simulink model "GRM_HIL"  (R2019b)
settings: Solver=FixedStepAuto  StartTime=0.0  StopTime=60  FixedStep=0.001  RelTol=1e-3
libraries: lib_GRM_HIL x7, simulink x1
settings Model: SimulationMode=external  Creator=m.hiepp  LastModifiedBy=guy-m
settings DataIOCC: SignalLogging=off  ReturnWorkspaceOutputs=off
settings DebuggingCC: ArithmeticOperatorsInVariantConditions=warning
settings SFSimCC: CustomCodeUndefinedFunction=UseInterfaceOnly
settings RTWCC: Description=Simulink Desktop Real-Time  SystemTargetFile=sldrt.tlc  TemplateMakefile=sldrt.tmf  RTWCompilerOptimization=on
settings CodeAppCC: MaxIdLength=95
settings SimulinkDesktopRealTimeCC: TargetPreCompLibLocation=C:\Program Files\MATLAB\R2019b\toolbox\sldrt\lib\win64  PreserveStateflowLocalDataDimensions=off

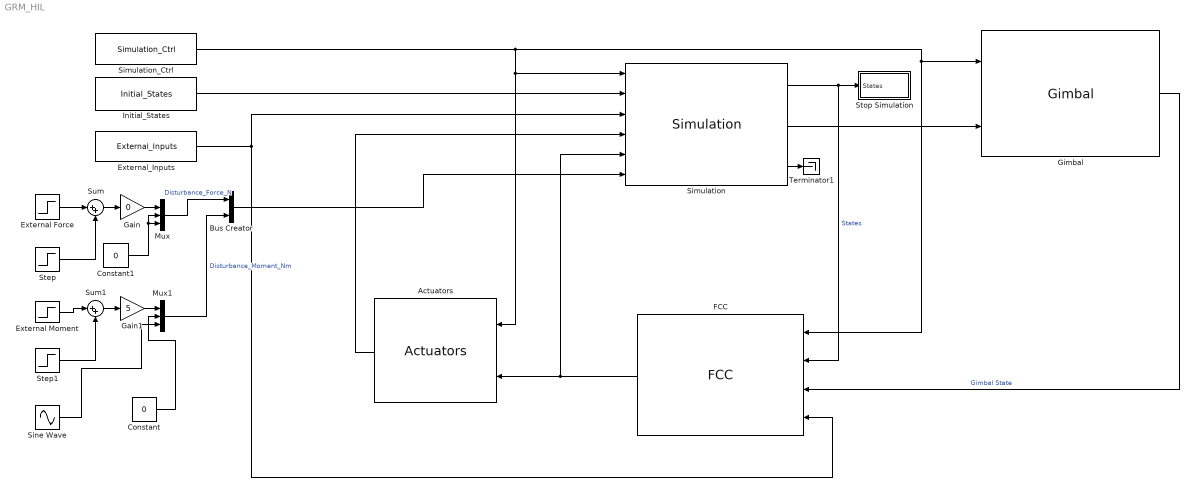
== system GRM_HIL ==
  Actuators : lib_GRM_HIL/Actuators  SystemSampleTime=-1  Latency=0  AutoFrameSizeCalculation=off
  Bus Creator : BusCreator  Inputs=2  OutDataTypeStr=Bus: Disturbances_Bus
  Constant : Constant  Value=0
  Constant1 : Constant  Value=0
  External Force : Step  Time=0  SampleTime=0
  External Moment : Step  Time=5  SampleTime=0
  External_Inputs : lib_GRM_HIL/External_Inputs  External_Inputs=HIL_Data.External_Inputs
  FCC : lib_GRM_HIL/FCC  SystemSampleTime=-1  Latency=0  AutoFrameSizeCalculation=off
      link override Use_FCC/Serial_Config_Pixhawk/enable_serial_config/Serial Configuration: ComPortMenu=COM4  BaudRate=115200  StopBits=1  ComPort=COM4  ObjConstructor=serial('COM4');
      link override Use_FCC/Serial_Recieve_from_Pixhawk/Receive_ExternalMode/Packet Input: SampleTime=HIL_Sample_Time  MaxMissedTicks=Serial.Receive.MaxMissedTicks  ShowMissedTicks=off  YieldWhenWaiting=on  DrvName=Standard_Devices/Serial_Port  DrvAddress=4  DrvOptions=[115200 8 0 0 0 0 0 0]  PacketSize=62  DataTypes='62*uint8'  ShowReady=on  ShowError=on  PacketID=1  ByteOrder=1  ShowTimestamp=off
      link override Use_FCC/Serial_Recieve_from_Pixhawk/Receive_NormalMode/Serial Configuration: ComPortMenu=COM4  BaudRate=115200  StopBits=1  ComPort=COM4  ObjConstructor=serial('COM4');
      link override Use_FCC/Serial_Recieve_from_Pixhawk/Receive_NormalMode/Serial Receive1: ComPortMenu=COM4  ComPort=COM4  ObjConstructor=serial('COM4');
      link override Use_FCC/Serial_Send_to_Pixhawk/send_to_pix/Send_ExternalMode/Packet Output: SampleTime=1/HIL_Data.Simulation_Ctrl.Com_Ctrl.Pix.Com_freq_Hz  MaxMissedTicks=Serial.Send.MaxMissedTicks  ShowMissedTicks=off  YieldWhenWaiting=on  DrvName=Standard_Devices/Serial_Port  DrvAddress=4  DrvOptions=[115200 8 0 0 0 0 0 0]  PacketSize=128  DataTypes='128*uint8'  ShowReady=off  ShowError=on  PacketID=1  ByteOrder=1  InitialValue=[]  FinalValue=[]
      link override Use_FCC/Serial_Send_to_Pixhawk/send_to_pix/Send_NormalMode/Packet Output: SampleTime=1/HIL_Data.Simulation_Ctrl.Com_Ctrl.Pix.Com_freq_Hz  MaxMissedTicks=Serial.Send.MaxMissedTicks  ShowMissedTicks=off  YieldWhenWaiting=on  DrvName=Standard_Devices/Serial_Port  DrvAddress=1  DrvOptions=[1152000 8 0 0 0 0 0 0]  PacketSize=128  DataTypes='128*uint8'  ShowReady=off  ShowError=on  PacketID=1  ByteOrder=1  InitialValue=[]  FinalValue=[]
  Gain : Gain  Gain=0
  Gain1 : Gain  Gain=5
  Gimbal : lib_GRM_HIL/Gimbal  SystemSampleTime=-1  Latency=0  AutoFrameSizeCalculation=off
      link override Use_Gimbal_HWInterface_CC/Communication_FT_HWI_ControlComputer/Construct_Bus/Assemble_Gimbal_Subbusses/Shaft2radPitch: Gain=-(2*pi)/(65536)
      link override Use_Gimbal_HWInterface_CC/Communication_FT_HWI_ControlComputer/Receive_from_FTHWICC: SampleTime=HW.SampTime  MaxMissedTicks=HW.MaxMissTick  ShowMissedTicks=off  YieldWhenWaiting=on  DrvName=Standard_Devices/UDP_Protocol  DrvAddress=36864  DrvOptions=[0 36880 49 46 49 46 49 46 49 0 0 0 0 0 0 0 0 0 0 0 0 0 0 0 0 0 0 0 0 0 0 0 0 0 0 0 0 0 0 0 0 0 0 0 0 0 0 0 0 0 0 0 0 0 0 0 0 0 0 0 0 0 0 0 0 0 0 0 0 0 0 0 0 0 0 0 0 0 0 0 0 0 0 0 0 0 0 0 0 0 0 0 0 0 0 0 0 0 0 0 0 0 0 0 0 0 0 0 0 0 0 0 0 0 0 0 0 0 0 0 0 0 0 0 0 0 0 0 0 0 0 0 0 0 0 0 0 0 0 0 0 0 0 0 0 0 0 0 0 0 0 0 0 0 0 0 0 0 0 0 0 0 0 0 0 0 0 0 0 0 0 0 0 0 0 0 0 0 0 0 0 0 0 0 0 0 0 0 0 0 0 0 0 0 0 0 0 0 0 0 0 0 0 0 0 0 0 0 0 0 0 0 0 0 0 0 0 0 0 0 0 0 0 0 0 0 0 0 0 0 0 0 0 0 0 0 0 0 0 0 0 0 0 0 0 0 0 0 0 0 0 0 0 0 0 0]  PacketSize=66  DataTypes={'double','double','double','double','double','double','double','uint16','double'}  ShowReady=on  ShowError=on  PacketID=1  ByteOrder=1  ShowTimestamp=off
      link override Use_Gimbal_HWInterface_CC/Communication_FT_HWI_ControlComputer/Send_to_FTHWICC/Send_to_FTHWICC: SampleTime=1/HIL_Data.Simulation_Ctrl.Com_Ctrl.FT.Com_freq_Hz  MaxMissedTicks=HW.MaxMissTick  ShowMissedTicks=off  YieldWhenWaiting=on  DrvName=Standard_Devices/UDP_Protocol  DrvAddress=36864  DrvOptions=[0 36880 49 46 49 46 49 46 49 0 0 0 0 0 0 0 0 0 0 0 0 0 0 0 0 0 0 0 0 0 0 0 0 0 0 0 0 0 0 0 0 0 0 0 0 0 0 0 0 0 0 0 0 0 0 0 0 0 0 0 0 0 0 0 0 0 0 0 0 0 0 0 0 0 0 0 0 0 0 0 0 0 0 0 0 0 0 0 0 0 0 0 0 0 0 0 0 0 0 0 0 0 0 0 0 0 0 0 0 0 0 0 0 0 0 0 0 0 0 0 0 0 0 0 0 0 0 0 0 0 0 0 0 0 0 0 0 0 0 0 0 0 0 0 0 0 0 0 0 0 0 0 0 0 0 0 0 0 0 0 0 0 0 0 0 0 0 0 0 0 0 0 0 0 0 0 0 0 0 0 0 0 0 0 0 0 0 0 0 0 0 0 0 0 0 0 0 0 0 0 0 0 0 0 0 0 0 0 0 0 0 0 0 0 0 0 0 0 0 0 0 0 0 0 0 0 0 0 0 0 0 0 0 0 0 0 0 0 0 0 0 0 0 0 0 0 0 0 0 0 0 0 0 0 0 0]  PacketSize=52  DataTypes={'boolean','boolean','double','double','uint16','double','double','double','double'}  ShowReady=off  ShowError=off  PacketID=1  ByteOrder=1  InitialValue=[]  FinalValue=[]
  Initial_States : lib_GRM_HIL/Initial_States  Rigid_Body=HIL_Data.Initial_States.Rigid_Body  Airframe=HIL_Data.Initial_States.Airframe  Atm=HIL_Data.Initial_States.Atm
  Mux : Mux  Inputs=3
  Mux1 : Mux  Inputs=3
  Simulation : lib_GRM_HIL/Simulation  SystemSampleTime=-1  Latency=0  AutoFrameSizeCalculation=off
  Simulation_Ctrl : lib_GRM_HIL/Simulation_Ctrl  SystemSampleTime=-1  Latency=0  AutoFrameSizeCalculation=off
  Sine Wave : Sin  Amplitude=5  Frequency=10  SampleTime=0
  Step : Step  Time=3  After=-1  SampleTime=0
  Step1 : Step  Time=6  After=-1  SampleTime=0
  Stop Simulation : Subsystem
  Sum : Sum  Inputs=|++
  Sum1 : Sum  Inputs=|++
  Terminator1 : Terminator
  wires:
  Gimbal/1 -> FCC/3  "Gimbal State"
  External_Inputs/1 -> FCC/4, Simulation/3
  Simulation_Ctrl/1 -> Gimbal/1, FCC/1, Actuators/1, Simulation/1
  Initial_States/1 -> Simulation/2
  Actuators/1 -> Simulation/4
  FCC/1 -> Simulation/5, Actuators/2
  External Force/1 -> Sum/1
  Step/1 -> Sum/2
  Sum/1 -> Gain/1
  Sum1/1 -> Gain1/1
  Step1/1 -> Sum1/2
  External Moment/1 -> Sum1/1
  Gain/1 -> Mux/1
  Gain1/1 -> Mux1/1
  Mux/1 -> Bus Creator/1  "Disturbance_Force_N"
  Mux1/1 -> Bus Creator/2  "Disturbance_Moment_Nm"
  Constant1/1 -> Mux/3, Mux/2
  Bus Creator/1 -> Simulation/6
  Simulation/1 -> FCC/2, Stop Simulation/1(States)  "States"
  Simulation/3 -> Terminator1/1
  Simulation/2 -> Gimbal/2
  Sine Wave/1 -> Mux1/3
  Constant/1 -> Mux1/2

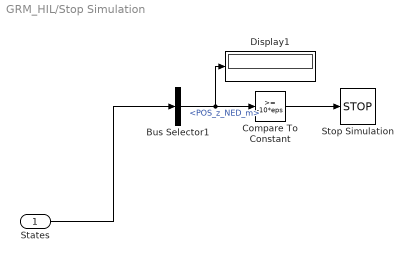
== system GRM_HIL/Stop Simulation ==
  States : Inport
  Bus Selector1 : BusSelector  OutputSignals=Rigid_Body_States.Position_States.POS_NED.POS_z_NED_m
  Compare To Constant : simulink/Logic and Bit Operations/Compare To Constant  relop=>=  const=-10*eps  OutDataTypeStr=boolean
  Display1 : Display
  Stop Simulation : Stop
  wires:
  Compare To Constant/1 -> Stop Simulation/1
  Bus Selector1/1 -> Display1/1, Compare To Constant/1  "<POS_z_NED_m>"
  States/1 -> Bus Selector1/1
